simulink model "LQR_Balancing_Robot"  (R2021b)
settings: Solver=FixedStepAuto  StartTime=0.0  StopTime=50  FixedStep=0.01  RelTol=1e-3
values from neighbouring files (symbols this model uses):
  K = lqr(A,B,Q,R)    [Ket_qua_LQR.m]
  x1_init = 0.001    [Ket_qua_LQR.m]
  x2_init = 0.001    [Ket_qua_LQR.m]
  x3_init = 0.002    [Ket_qua_LQR.m]
  x4_init = 0.002    [Ket_qua_LQR.m]
  x5_init = 0.002    [Ket_qua_LQR.m]
  x6_init = 0.003    [Ket_qua_LQR.m]
settings Model: Creator=toani  LastModifiedBy=toani
settings DataIOCC: ReturnWorkspaceOutputs=off  LoggingToFile=on

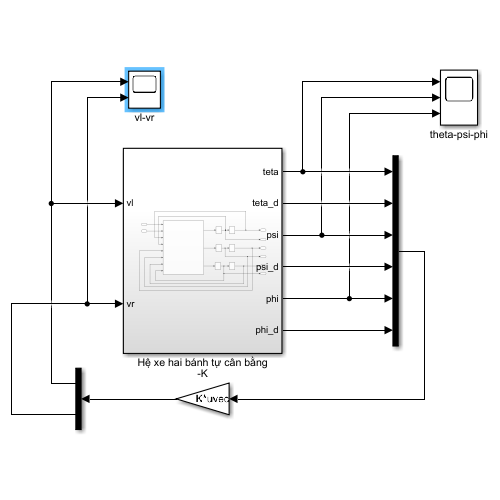
[thumbnail: Simulink's stored preview of the top-level diagram]
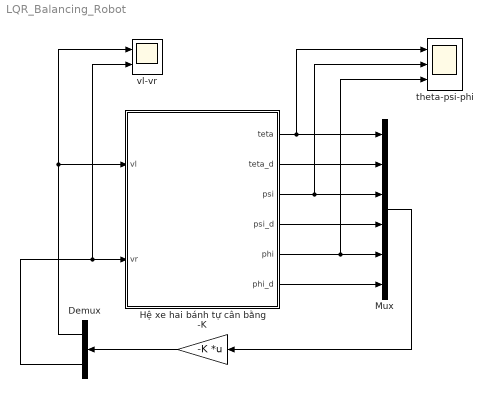
== system LQR_Balancing_Robot ==
  -K : Gain  Gain=-K  Multiplication=Matrix(K*u) (u vector)
  Demux : Demux  Outputs=2
  Hệ xe hai bánh tự cân bằng : Subsystem
  Mux : Mux  Inputs=6
  theta-psi-phi : Scope  NumInputPorts=3
  vl-vr : Scope  NumInputPorts=2
  wires:
  Hệ xe hai bánh tự cân bằng/1(teta) -> theta-psi-phi/1, Mux/1
  Hệ xe hai bánh tự cân bằng/2(teta_d) -> Mux/2
  Hệ xe hai bánh tự cân bằng/3(psi) -> theta-psi-phi/2, Mux/3
  Hệ xe hai bánh tự cân bằng/4(psi_d) -> Mux/4
  Hệ xe hai bánh tự cân bằng/5(phi) -> theta-psi-phi/3, Mux/5
  Hệ xe hai bánh tự cân bằng/6(phi_d) -> Mux/6
  Mux/1 -> -K/1
  -K/1 -> Demux/1
  Demux/1 -> vl-vr/1, Hệ xe hai bánh tự cân bằng/1(vl)
  Demux/2 -> vl-vr/2, Hệ xe hai bánh tự cân bằng/2(vr)

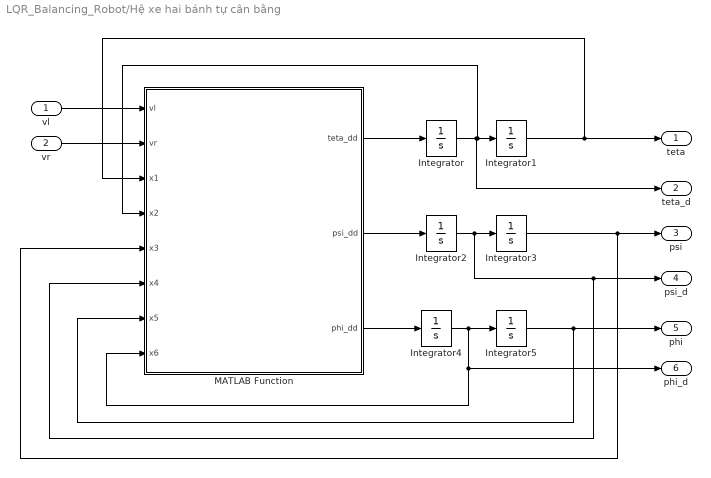
== system LQR_Balancing_Robot/Hệ xe hai bánh tự cân bằng ==
  vl : Inport
  vr : Inport  Port=2
  Integrator : Integrator  InitialCondition=x2_init
  Integrator1 : Integrator  InitialCondition=x1_init
  Integrator2 : Integrator  InitialCondition=x4_init
  Integrator3 : Integrator  InitialCondition=x3_init
  Integrator4 : Integrator  InitialCondition=x6_init
  Integrator5 : Integrator  InitialCondition=x5_init
  MATLAB Function : MATLAB Function  TreatAsAtomicUnit=on
  teta : Outport
  teta_d : Outport  Port=2
  psi : Outport  Port=3
  psi_d : Outport  Port=4
  phi : Outport  Port=5
  phi_d : Outport  Port=6
  wires:
  Integrator5/1 -> phi/1, MATLAB Function/7(x5)
  vr/1 -> MATLAB Function/2(vr)
  Integrator4/1 -> phi_d/1, MATLAB Function/8(x6), Integrator5/1
  MATLAB Function/3(phi_dd) -> Integrator4/1
  Integrator2/1 -> psi_d/1, MATLAB Function/6(x4), Integrator3/1
  MATLAB Function/2(psi_dd) -> Integrator2/1
  Integrator/1 -> teta_d/1, MATLAB Function/4(x2), Integrator1/1
  Integrator1/1 -> teta/1, MATLAB Function/3(x1)
  Integrator3/1 -> psi/1, MATLAB Function/5(x3)
  vl/1 -> MATLAB Function/1(vl)
  MATLAB Function/1(teta_dd) -> Integrator/1

== matlab function LQR_Balancing_Robot/Hệ xe hai bánh tự cân bằng/MATLAB Function ==
  data: vl input; teta_dd output; vr input; x1 input; x2 input; x3 input; x4 input; x5 input; x6 input; psi_dd output; phi_dd output
function [teta_dd,psi_dd,phi_dd] = system(vl,vr,x1,x2,x3,x4,x5,x6)
%% Thông số hệ thống xe 2 bánh tự cân bằng dùng LQR
m = 0.042; %Khoi luong banh xe
M = 1.08; %Khoi luong robot
R = 0.0325; %ban kinh ban xe
W = 0.170; %Chieu rong robot
D = 0.100; %Chieu ngang robot
H = 0.1415; %Chieu cao robot
L = H/2; %khoang cach tu trong tam den truc banh xe
fw = 0.18; %He so ma sat giua banh xe voi mat phang
fm = 0.002; %he so ma sat giua dong co va robot
Jm = 0.01; %moment quan tinh cua dong co
Jw = m*R^2/2;
J_psi = 2*M*L^2/3;
J_phi = M*(W^2+D^2)/12;
Rm = 50; %Dien tro dong co DC
Kb = 0.468; %he so emf cua dong co
Kt = 0.317; %Momen xoan cua dong co DC
n = 30; %Ty so giam toc
g = 9.81; %Gia toc trong truong
alpha = n*Kt/Rm; beta=n*Kt*Kb/Rm+fm; a =alpha;
%T=0.01;
%% Cac phuong trinh vi phan
teta_dd = (J_psi*a*vl + J_psi*a*vr - 2*J_psi*beta*x2 + 2*J_psi*beta*x4 - 2*J_psi*fw*x2 + L^2*M*a*vl + L^2*M*a*vr - 2*L^2*M*beta*x2 + 2*L^2*M*beta*x4 - 2*L^2*M*fw*x2 - 4*Jm*fw*n^2*x2 - (L^2*M^2*R*g*sin(2*x3))/2 + L^3*M^2*R*x4^2*sin(x3) - L^3*M^2*R*x6^2*(sin(x3) - sin(x3)^3) - 2*L*M*R*beta*x2*cos(x3) + 2*L*M*R*beta*x4*cos(x3) + J_psi*L*M*R*x4^2*sin(x3) + 2*Jm*L*M*g*n^2*sin(x3) + Jm*L^2*M*n^2*x6^2*sin(2*x3) + L*M*R*a*vl*cos(x3) + L*M*R*a*vr*cos(x3) + 2*Jm*L*M*R*n^2*x4^2*sin(x3))/(2*J_psi*Jw + L^2*M^2*R^2 + 2*Jw*L^2*M + J_psi*M*R^2 + 2*J_psi*Jm*n^2 + 4*Jm*Jw*n^2 + 2*J_psi*R^2*m + 2*Jm*L^2*M*n^2 + 2*Jm*M*R^2*n^2 + 2*L^2*M*R^2*m + 4*Jm*R^2*m*n^2 - L^2*M^2*R^2*cos(x3)^2 + 4*Jm*L*M*R*n^2*cos(x3));
psi_dd = -(2*Jw*a*vl + 2*Jw*a*vr - 4*Jw*beta*x2 + 4*Jw*beta*x4 + M*R^2*a*vl + M*R^2*a*vr - 2*M*R^2*beta*x2 + 2*M*R^2*beta*x4 + 2*R^2*a*m*vl + 2*R^2*a*m*vr + 4*Jm*fw*n^2*x2 - 4*R^2*beta*m*x2 + 4*R^2*beta*m*x4 - L*M^2*R^2*g*sin(x3) + (L^2*M^2*R^2*x4^2*sin(2*x3))/2 - (L^2*M^2*R^2*x6^2*sin(2*x3))/2 - 2*Jw*L*M*g*sin(x3) - Jw*L^2*M*x6^2*sin(2*x3) - 2*L*M*R*beta*x2*cos(x3) + 2*L*M*R*beta*x4*cos(x3) - 2*L*M*R*fw*x2*cos(x3) - 2*Jm*L*M*g*n^2*sin(x3) - 2*L*M*R^2*g*m*sin(x3) - Jm*L^2*M*n^2*x6^2*sin(2*x3) - L^2*M*R^2*m*x6^2*sin(2*x3) + L*M*R*a*vl*cos(x3) + L*M*R*a*vr*cos(x3) - 2*Jm*L*M*R*n^2*x4^2*sin(x3))/(2*J_psi*Jw + L^2*M^2*R^2 + 2*Jw*L^2*M + J_psi*M*R^2 + 2*J_psi*Jm*n^2 + 4*Jm*Jw*n^2 + 2*J_psi*R^2*m + 2*Jm*L^2*M*n^2 + 2*Jm*M*R^2*n^2 + 2*L^2*M*R^2*m + 4*Jm*R^2*m*n^2 - L^2*M^2*R^2*cos(x3)^2 + 4*Jm*L*M*R*n^2*cos(x3));
phi_dd = -(W^2*beta*x6 + W^2*fw*x6 + R*W*a*vl - R*W*a*vr + 2*L^2*M*R^2*x4*x6*sin(2*x3))/(2*J_phi*R^2 + Jw*W^2 + Jm*W^2*n^2 + R^2*W^2*m + 2*L^2*M*R^2*sin(x3)^2); 
end
